simulink model "Mdl_Dim"  (R2024b)
settings: Solver=FixedStepDiscrete  StartTime=0.0  StopTime=10.0  FixedStep=0.1  RelTol=1e-3  EnableMultiTasking=on
values from neighbouring files (symbols this model uses):
  DEFAULT_MODE = mpt.Parameter    [Mdl_Dim_DD.m]
  DEFAULT_STEP = mpt.Parameter    [Mdl_Dim_DD.m]
  Mdl_Dim_cTaskPeriod = mpt.Parameter    [Mdl_Dim_rte_types.m]
  RTE_E_MAX_AGE_EXCEEDED = mpt.Parameter    [Mdl_Dim_rte_types.m]
  RTE_E_NEVER_RECEIVED = mpt.Parameter    [Mdl_Dim_rte_types.m]
  STATUS_OFF = mpt.Parameter    [Mdl_Dim_DD.m]
  STATUS_ON = mpt.Parameter    [Mdl_Dim_DD.m]
  SWITCHING_MECHANISM = mpt.Parameter    [Mdl_Dim_DD.m]
  ZERO_VAL = mpt.Parameter    [Mdl_Dim_DD.m]
undefined symbols (not defined in the file or in its folder): AppModule, CAN_COMUN_ACTIVE, CAN_COMUN_FAIL, CAN_VAL_OFF, CAN_VAL_ON, ChannelID, CLUSTER_ACTIVE, DAYNIGHT_STS_NOTRequire, DIAG_NCTRL, DIM_DAY_MODE, DIM_NIGHT_MODE, DOWN_THRESH_1SW, DrvRec_Rheo_down_Long_Press, DrvRec_Rheo_down_Short_Press, DrvRec_Rheo_up_Long_Press, DrvRec_Rheo_Up_Short_Press, DW_EVENT, DW_ON, eAppMdl_type_instance, eDayNightModeIn, eIllumination_levelIn, eSIGNAL_MISSING, eSIGNAL_NEVER_RECEIVED, eSleepSt_type_instance, FALSE, GetPwmDirect, GetPwmWithTime, GetPwmWithTimeExp, IgnOn, INDEX_MCUID0340, INDEX_MCUID0341, INDEX_MCUID0430, IoHwAb_PwmSignalIdType_type_instance, l_Wheel_Down_ParamArray, l_Wheel_Up_ParamArray, MAX_UINT16, MAXHOLD, MINHOLD, NETWORK_NORMAL, NETWORK_SLEEP, NETWORK_STANDALONE, NONE, NVM_Adapter_SetNVM_RheostatDayStep, NVM_Adapter_SetNVM_RheostatDayStepU1, NVM_Adapter_SetNVM_RheostatDayStepU2, NVM_Adapter_SetNVM_RheostatDayStepU3, NVM_Adapter_SetNVM_RheostatNightStep, NVM_Adapter_SetNVM_RheostatNightStepU1, NVM_Adapter_SetNVM_RheostatNightStepU2, NVM_Adapter_SetNVM_RheostatNightStepU3, OpeModeRheostatChange, pJustRcvdStatus, pNvmData, POS_MAX, POS_MIN, RHEO_1SW_TYPE, RHEO_2SW_TYPE, RHEO_SOFTSW_TYPE, RHEO_VALUE_FIVE_U16, RHEO_VALUE_ONE_BOOL ... (+48)
libraries: simulink x65
(part 3 of 4)

== system Mdl_Dim/Mdl_Dim_Task_sys/Subsystem/Input_Process/Switch Type//2 Switch Type//Soft Switch Type/RHEO_1SW_TYPE_AND_RHEO_2SW_TYPE/Subsystem2 ==
  ADC_RHDW_val : Inport
  AND : Logic  AllPortsSameDT=off  OutDataTypeStr=boolean
  Compare To Constant : simulink/Logic and Bit Operations/Compare To Constant  relop=~=  const=RHEO_VALUE_ZERO_BOOL  OutDataTypeStr=boolean
  Compare To Constant1 : simulink/Logic and Bit Operations/Compare To Constant  relop=~=  const=RHEO_VALUE_ONE_BOOL  OutDataTypeStr=boolean
  Compare To Constant5 : simulink/Logic and Bit Operations/Compare To Constant  relop===  const=RHEO_VALUE_ONE_BOOL  OutDataTypeStr=boolean
  Constant4 : Constant  Value=RHEO_VALUE_ONE_U16  OutDataTypeStr=Inherit: Inherit via back propagation
  Constant5 : Constant  Value=RHEO_VALUE_ZERO_U16  OutDataTypeStr=Inherit: Inherit via back propagation
  Constant6 : Constant  Value=RHEO_VALUE_ZERO_U16  OutDataTypeStr=uint16
  Constant7 : Constant  Value=RHEO_VALUE_FIVE_U16  OutDataTypeStr=Inherit: Inherit via back propagation
  Subtract1 : Sum  Inputs=+-
  Switch2 : Switch  Criteria=u2 ~= 0  OutDataTypeStr=uint16  SaturateOnIntegerOverflow=off  InputSameDT=off
  Switch3 : Switch  Criteria=u2 ~= 0  OutDataTypeStr=uint16  RndMeth=Simplest  SaturateOnIntegerOverflow=off  InputSameDT=off
  Unit Delay : UnitDelay  SampleTime=-1  StateName=Prev_RHDW_RawIn_Val  HasFrameUpgradeWarning=on
  Unit Delay2 : UnitDelay  InitialCondition=ZERO_DUTY  SampleTime=-1  StateName=Prev_SW1Rheostat_Dw_time_Step50ms  HasFrameUpgradeWarning=on
  check count2 : RelationalOperator  Operator=~=  OutDataTypeStr=boolean  InputSameDT=off
  RHDW_RawIn_Val_50ms : Outport  VectorParamsAs1DForOutWhenUnconnected=off
  wires:
  Unit Delay2/1 -> Switch2/3  "current_count_2"
  Switch2/1 -> Subtract1/1, check count2/1  "current_count_2"
  check count2/1 -> RHDW_RawIn_Val_50ms/1, Switch3/2  "fl_RHDW_RawIn_Val_50ms"
  Compare To Constant5/1 -> Switch2/2
  Constant4/1 -> Subtract1/2  "Decrement_Value_2"
  Constant7/1 -> Switch2/1  "Decrement_Value_DW"
  Switch3/1 -> Unit Delay2/1
  Constant5/1 -> check count2/2  "Max_step_Count2"
  ADC_RHDW_val/1 -> [RHDW_RawIn_Val], Unit Delay/1
  Unit Delay/1 -> [Prev_RHDW_RawIn_Val]
  [RHDW_RawIn_Val] -> Compare To Constant/1
  [Prev_RHDW_RawIn_Val] -> Compare To Constant1/1
  Constant6/1 -> Switch3/3
  Subtract1/1 -> Switch3/1  "current_count_2"
  Compare To Constant/1 -> AND/1
  Compare To Constant1/1 -> AND/2
  AND/1 -> Compare To Constant5/1

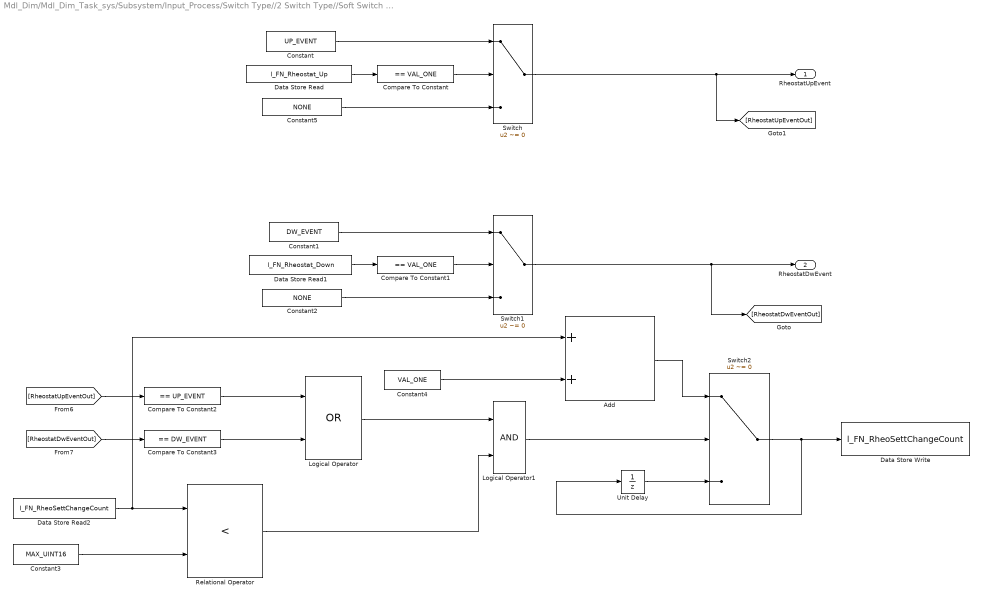
== system Mdl_Dim/Mdl_Dim_Task_sys/Subsystem/Input_Process/Switch Type//2 Switch Type//Soft Switch Type/Soft Switch Type/Event Check ==
  Add : Sum
  Compare To Constant : simulink/Logic and Bit Operations/Compare To Constant  relop===  const=VAL_ONE  OutDataTypeStr=boolean
  Compare To Constant1 : simulink/Logic and Bit Operations/Compare To Constant  relop===  const=VAL_ONE  OutDataTypeStr=boolean
  Compare To Constant2 : simulink/Logic and Bit Operations/Compare To Constant  relop===  const=UP_EVENT  OutDataTypeStr=boolean
  Compare To Constant3 : simulink/Logic and Bit Operations/Compare To Constant  relop===  const=DW_EVENT  OutDataTypeStr=boolean
  Constant : Constant  Value=UP_EVENT
  Constant1 : Constant  Value=DW_EVENT
  Constant2 : Constant  Value=NONE
  Constant3 : Constant  Value=MAX_UINT16  OutDataTypeStr=uint16
  Constant4 : Constant  Value=VAL_ONE  OutDataTypeStr=uint16
  Constant5 : Constant  Value=NONE
  Data Store Read : DataStoreRead  DataStoreName=l_FN_Rheostat_Up  IndexOptions=Index vector (dialog)  Indices=1  OutputSizes=1
  Data Store Read1 : DataStoreRead  DataStoreName=l_FN_Rheostat_Down  IndexOptions=Index vector (dialog)  Indices=1  OutputSizes=1
  Data Store Read2 : DataStoreRead  DataStoreName=l_FN_RheoSettChangeCount  IndexOptions=Index vector (dialog)  Indices=1  OutputSizes=1
  Data Store Write : DataStoreWrite  DataStoreName=l_FN_RheoSettChangeCount  IndexOptions=Index vector (dialog)  Indices=1  OutputSizes=1
  Logical Operator : Logic  Operator=OR  AllPortsSameDT=off  OutDataTypeStr=boolean
  Logical Operator1 : Logic  AllPortsSameDT=off  OutDataTypeStr=boolean
  Relational Operator : RelationalOperator  Operator=<  OutDataTypeStr=boolean  RndMeth=Simplest  InputSameDT=off
  Switch : Switch  Criteria=u2 ~= 0  SaturateOnIntegerOverflow=off  InputSameDT=off
  Switch1 : Switch  Criteria=u2 ~= 0  SaturateOnIntegerOverflow=off  InputSameDT=off
  Switch2 : Switch  Criteria=u2 ~= 0  SaturateOnIntegerOverflow=off  InputSameDT=off
  Unit Delay : UnitDelay  SampleTime=-1  HasFrameUpgradeWarning=on
  RheostatUpEvent : Outport  VectorParamsAs1DForOutWhenUnconnected=off
  RheostatDwEvent : Outport  Port=2  VectorParamsAs1DForOutWhenUnconnected=off
  wires:
  Compare To Constant1/1 -> Switch1/2
  Constant/1 -> Switch/1
  Data Store Read1/1 -> Compare To Constant1/1
  Data Store Read/1 -> Compare To Constant/1
  Constant1/1 -> Switch1/1
  Compare To Constant/1 -> Switch/2
  Constant2/1 -> Switch1/3
  Constant5/1 -> Switch/3
  Switch1/1 -> [RheostatDwEventOut], RheostatDwEvent/1
  Switch/1 -> [RheostatUpEventOut], RheostatUpEvent/1
  Switch2/1 -> Unit Delay/1, Data Store Write/1
  Data Store Read2/1 -> Add/1, Relational Operator/1
  [RheostatDwEventOut] -> Compare To Constant3/1
  Constant4/1 -> Add/2
  Relational Operator/1 -> Logical Operator1/2
  Unit Delay/1 -> Switch2/3
  Logical Operator/1 -> Logical Operator1/1
  Constant3/1 -> Relational Operator/2
  Add/1 -> Switch2/1
  [RheostatUpEventOut] -> Compare To Constant2/1
  Compare To Constant2/1 -> Logical Operator/1
  Compare To Constant3/1 -> Logical Operator/2
  Logical Operator1/1 -> Switch2/2

== system Mdl_Dim/Mdl_Dim_Task_sys/Subsystem/Input_Process/Switch Type//2 Switch Type//Soft Switch Type/Soft Switch Type/Event Clear ==
  Constant3 : Constant  Value=NONE
  Constant4 : Constant  Value=NONE
  Data Store Write : DataStoreWrite  DataStoreName=l_FN_Rheostat_Up  IndexOptions=Index vector (dialog)  Indices=1  OutputSizes=1
  Data Store Write1 : DataStoreWrite  DataStoreName=l_FN_Rheostat_Down  IndexOptions=Index vector (dialog)  Indices=1  OutputSizes=1
  wires:
  Constant3/1 -> Data Store Write/1
  Constant4/1 -> Data Store Write1/1

== system Mdl_Dim/Mdl_Dim_Task_sys/Subsystem/Input_Process/Switch Type//2 Switch Type//Soft Switch Type/Subsystem1/If Action Subsystem ==
  Action Port : ActionPort
  Constant : Constant  Value=VAL_ON
  Data Store Read1 : DataStoreRead  DataStoreName=l_Prev_NVM_RheostatNightStep  IndexOptions=Index vector (dialog)  Indices=1  OutputSizes=1
  Data Store Read2 : DataStoreRead  DataStoreName=l_Prev_NVM_RheostatDayStep  IndexOptions=Index vector (dialog)  Indices=1  OutputSizes=1
  NVM_Adapter_SetNVM_RheostatDayStep : FunctionCaller  FunctionPrototype=NVM_Adapter_SetNVM_RheostatDayStep(pNvmData)  InputArgumentSpecifications=uint8(1)  OutputArgumentSpecifications=<Enter example>
  NVM_Adapter_SetNVM_RheostatNightStep : FunctionCaller  FunctionPrototype=NVM_Adapter_SetNVM_RheostatNightStep(pNvmData)  InputArgumentSpecifications=uint8(1)  OutputArgumentSpecifications=<Enter example>
  OpeModeRheostatChange : FunctionCaller  FunctionPrototype=OpeModeRheostatChange()  InputArgumentSpecifications=<Enter example>  OutputArgumentSpecifications=<Enter example>
  RheostatChange : Outport  VectorParamsAs1DForOutWhenUnconnected=off
  wires:
  Constant/1 -> RheostatChange/1
  Data Store Read1/1 -> NVM_Adapter_SetNVM_RheostatNightStep/1
  Data Store Read2/1 -> NVM_Adapter_SetNVM_RheostatDayStep/1

== system Mdl_Dim/Mdl_Dim_Task_sys/Subsystem/Input_Process/Switch Type//2 Switch Type//Soft Switch Type/Subsystem1/If Action Subsystem1 ==
  Action Port : ActionPort
  Constant : Constant  Value=VAL_OFF
  RheostatChange : Outport  VectorParamsAs1DForOutWhenUnconnected=off
  wires:
  Constant/1 -> RheostatChange/1

== system Mdl_Dim/Mdl_Dim_Task_sys/Subsystem/Input_Process/Thumb Wheel Type/Rheostat_ONS_Status_Output /Debounce_timer_Subsystem2 ==
  Debounce_Count : Inport
  "ResetTimerStatus " : Inport  Port=2
  Compare To Zero : simulink/Logic and Bit Operations/Compare To Zero  relop=~=  OutDataTypeStr=boolean
  Compare To Zero1 : simulink/Logic and Bit Operations/Compare To Zero  relop=~=  OutDataTypeStr=boolean
  Constant1 : Constant  Value=VAL_ONE  OutDataTypeStr=uint8
  Constant2 : Constant  Value=VAL_ONE  OutDataTypeStr=uint8
  Constant3 : Constant  Value=VAL_ZERO  OutDataTypeStr=uint8
  Constant4 : Constant  Value=VAL_ZERO  OutDataTypeStr=uint8
  Data Store Read : DataStoreRead  DataStoreName=l_Prev_Rheo3secCount  IndexOptions=Index vector (dialog)  Indices=1  OutputSizes=1
  Data Store Read1 : DataStoreRead  DataStoreName=l_Prev_Rheo3secCount  IndexOptions=Index vector (dialog)  Indices=1  OutputSizes=1
  Data Store Write : DataStoreWrite  DataStoreName=l_Prev_Rheo3secCount  IndexOptions=Index vector (dialog)  Indices=1  OutputSizes=1
  Sum : Sum
  Switch1 : Switch  Criteria=u2 ~= 0  OutDataTypeStr=uint32  SaturateOnIntegerOverflow=off  InputSameDT=off
  Switch2 : Switch  Criteria=u2 ~= 0  OutDataTypeStr=uint32  SaturateOnIntegerOverflow=off  InputSameDT=off
  Switch3 : Switch  Criteria=u2 ~= 0  OutDataTypeStr=uint32  SaturateOnIntegerOverflow=off  InputSameDT=off
  check count1 : RelationalOperator  Operator=<=  OutDataTypeStr=boolean  InputSameDT=off
  wires:
  "ResetTimerStatus "/1 -> Compare To Zero/1
  Switch2/1 -> Switch3/3, check count1/2  "current_count"
  Debounce_Count/1 -> check count1/1  "debounce_count"
  check count1/1 -> Switch3/2  "debounce_status"
  Constant2/1 -> Switch2/1
  Compare To Zero/1 -> Switch2/2
  Constant1/1 -> Sum/1
  Data Store Read/1 -> Sum/2
  Data Store Read1/1 -> Compare To Zero1/1
  Compare To Zero1/1 -> Switch1/2
  Switch1/1 -> Switch2/3
  Sum/1 -> Switch1/1
  Constant3/1 -> Switch1/3
  Switch3/1 -> Data Store Write/1
  Constant4/1 -> Switch3/1

== system Mdl_Dim/Mdl_Dim_Task_sys/Subsystem/Input_Process/Thumb Wheel Type/Rheostat_ONS_Status_Output /Subsystem3 ==
  Action Port : ActionPort
  Constant : Constant  Value=VAL_ONE
  Data Store Write : DataStoreWrite  DataStoreName=RheostatONSStatus  IndexOptions=Index vector (dialog)  Indices=1  OutputSizes=1
  wires:
  Constant/1 -> Data Store Write/1

== system Mdl_Dim/Mdl_Dim_Task_sys/Subsystem/Input_Process/Thumb Wheel Type/Rheostat_ONS_Status_Output /Subsystem4 ==
  Action Port : ActionPort
  Constant1 : Constant  Value=VAL_TWO
  Data Store Write : DataStoreWrite  DataStoreName=RheostatONSStatus  IndexOptions=Index vector (dialog)  Indices=1  OutputSizes=1
  wires:
  Constant1/1 -> Data Store Write/1

== system Mdl_Dim/Mdl_Dim_Task_sys/Subsystem/Input_Process/Thumb Wheel Type/Rheostat_ONS_Status_Output /Subsystem5 ==
  Action Port : ActionPort
  Constant1 : Constant  Value=VAL_ZERO
  Data Store Read : DataStoreRead  DataStoreName=RheostatONSStatus  IndexOptions=Index vector (dialog)  Indices=1  OutputSizes=1
  Data Store Read1 : DataStoreRead  DataStoreName=l_Prev_Rheo3secCount  IndexOptions=Index vector (dialog)  Indices=1  OutputSizes=1
  Data Store Write : DataStoreWrite  DataStoreName=RheostatONSStatus  IndexOptions=Index vector (dialog)  Indices=1  OutputSizes=1
  Switch : Switch  Criteria=u2 ~= 0  SaturateOnIntegerOverflow=off  InputSameDT=off
  wires:
  Data Store Read1/1 -> Switch/2
  Constant1/1 -> Switch/3
  Switch/1 -> Data Store Write/1
  Data Store Read/1 -> Switch/1

== system Mdl_Dim/Mdl_Dim_Task_sys/Subsystem/Input_Process/Thumb Wheel Type/Subsystem/Subsystem1 ==
  RHEO_SW_WHEEL : Inport
  ADC_RHEO_5V_MON_ADI : Inport  Port=2
  Compare To Constant : simulink/Logic and Bit Operations/Compare To Constant  relop=>=  const=WHEELVOLRATIO_SAMPLE_COUNT  OutDataTypeStr=boolean
  Data Store Read1 : DataStoreRead  DataStoreName=l_Wheel_Vol_Counter_u8  IndexOptions=Index vector (dialog)  Indices=1  OutputSizes=1
  Enabled Subsystem : Subsystem  TreatAsAtomicUnit=on
  Subsystem : Subsystem
  wires:
  Data Store Read1/1 -> Compare To Constant/1
  Compare To Constant/1 -> Enabled Subsystem/Enable
  ADC_RHEO_5V_MON_ADI/1 -> Subsystem/2(ADC_RHEO_5V_MON_ADI)
  RHEO_SW_WHEEL/1 -> Subsystem/1(RHEO_SW_WHEEL)

== system Mdl_Dim/Mdl_Dim_Task_sys/Subsystem/Input_Process/Switch Type//2 Switch Type//Soft Switch Type/RHEO_1SW_TYPE_AND_RHEO_2SW_TYPE/ Rheostat Dw  Event Determination/Enabled Subsystem ==
  Enable : EnablePort
  Constant : Constant  OutDataTypeStr=boolean
  DrvRec_Rheo_down_Long_Press : FunctionCaller  FunctionPrototype=DrvRec_Rheo_down_Long_Press(SWGrp4LongPress_Status)  InputArgumentSpecifications=boolean(1)  OutputArgumentSpecifications=<Enter example>
  wires:
  Constant/1 -> DrvRec_Rheo_down_Long_Press/1

== system Mdl_Dim/Mdl_Dim_Task_sys/Subsystem/Input_Process/Switch Type//2 Switch Type//Soft Switch Type/RHEO_1SW_TYPE_AND_RHEO_2SW_TYPE/ Rheostat Dw  Event Determination/Enabled Subsystem1 ==
  Enable : EnablePort
  Constant : Constant  OutDataTypeStr=boolean
  DrvRec_Rheo_down_Short_Press : FunctionCaller  FunctionPrototype=DrvRec_Rheo_down_Short_Press(SWGrp4ShortPress_Status)  InputArgumentSpecifications=boolean(1)  OutputArgumentSpecifications=<Enter example>
  wires:
  Constant/1 -> DrvRec_Rheo_down_Short_Press/1

== system Mdl_Dim/Mdl_Dim_Task_sys/Subsystem/Input_Process/Switch Type//2 Switch Type//Soft Switch Type/RHEO_1SW_TYPE_AND_RHEO_2SW_TYPE/ Rheostat Dw  Event Determination/Timer_100ms ==
  Debounce_Count : Inport
  "ResetTimerStatus " : Inport  Port=2
  Timer_In : Inport  Port=3
  Compare To Zero : simulink/Logic and Bit Operations/Compare To Zero  relop===  OutDataTypeStr=boolean
  Constant1 : Constant  Value=VAL_ONE  OutDataTypeStr=uint8
  Constant2 : Constant  Value=VAL_ZERO  OutDataTypeStr=uint8
  OR : Logic  Operator=OR  AllPortsSameDT=off  OutDataTypeStr=boolean
  Sum : Sum
  Switch2 : Switch  Criteria=u2 ~= 0  OutDataTypeStr=uint16  SaturateOnIntegerOverflow=off  InputSameDT=off
  check count1 : RelationalOperator  Operator=<=  OutDataTypeStr=boolean  InputSameDT=off
  TimerDebouncestatus : Outport  VectorParamsAs1DForOutWhenUnconnected=off
  Timer_out : Outport  Port=2  VectorParamsAs1DForOutWhenUnconnected=off
  wires:
  "ResetTimerStatus "/1 -> Compare To Zero/1
  Constant2/1 -> Switch2/1
  Sum/1 -> Switch2/3, check count1/2
  Constant1/1 -> Sum/1
  check count1/1 -> OR/2, TimerDebouncestatus/1  "debounce_status"
  Debounce_Count/1 -> [Debounce_Count]  "debounce_count"
  [Debounce_Count] -> check count1/1
  Compare To Zero/1 -> OR/1
  OR/1 -> Switch2/2
  Switch2/1 -> Timer_out/1  "current_count"
  Timer_In/1 -> Sum/2

== system Mdl_Dim/Mdl_Dim_Task_sys/Subsystem/Input_Process/Switch Type//2 Switch Type//Soft Switch Type/RHEO_1SW_TYPE_AND_RHEO_2SW_TYPE/ Rheostat Dw  Event Determination/Timer_800ms ==
  Debounce_Count : Inport
  "ResetTimerStatus " : Inport  Port=2
  l_PrevTimerSt_In : Inport  Port=3
  AND : Logic  AllPortsSameDT=off  OutDataTypeStr=boolean
  Constant1 : Constant  Value=VAL_ONE  OutDataTypeStr=uint8
  Constant2 : Constant  Value=VAL_ZERO  OutDataTypeStr=uint8
  Constant3 : Constant  Value=VAL_ZERO  OutDataTypeStr=uint8
  Sum : Sum
  Switch2 : Switch  Criteria=u2 ~= 0  OutDataTypeStr=uint32  SaturateOnIntegerOverflow=off  InputSameDT=off
  Switch3 : Switch  Criteria=u2 ~= 0  OutDataTypeStr=uint16  SaturateOnIntegerOverflow=off  InputSameDT=off
  check count : RelationalOperator  OutDataTypeStr=boolean  InputSameDT=off
  check count1 : RelationalOperator  Operator=~=  OutDataTypeStr=boolean  InputSameDT=off
  check count2 : RelationalOperator  Operator=>  OutDataTypeStr=boolean  InputSameDT=off
  Timer_800ms_elapsed_status : Outport  VectorParamsAs1DForOutWhenUnconnected=off
  Timer_Running_Status : Outport  Port=2  VectorParamsAs1DForOutWhenUnconnected=off
  l_PrevTimerSt_Out : Outport  Port=3  VectorParamsAs1DForOutWhenUnconnected=off
  wires:
  "ResetTimerStatus "/1 -> Switch2/2
  Switch2/1 -> Switch3/3, check count/1  "current_count"
  Debounce_Count/1 -> check count/2, check count2/1, Switch3/1  "debounce_count"
  check count/1 -> Timer_800ms_elapsed_status/1, Switch3/2  "debounce_status"
  Switch3/1 -> l_PrevTimerSt_Out/1
  Constant2/1 -> Switch2/1
  Sum/1 -> Switch2/3
  l_PrevTimerSt_In/1 -> check count1/2, check count2/2, Sum/2
  Constant1/1 -> Sum/1
  Constant3/1 -> check count1/1
  check count2/1 -> AND/1  "debounce_status"
  check count1/1 -> AND/2  "debounce_status"
  AND/1 -> Timer_Running_Status/1

== system Mdl_Dim/Mdl_Dim_Task_sys/Subsystem/Input_Process/Switch Type//2 Switch Type//Soft Switch Type/RHEO_1SW_TYPE_AND_RHEO_2SW_TYPE/ Rheostat Up Event Determination/Enabled Subsystem ==
  Enable : EnablePort
  Constant : Constant  OutDataTypeStr=boolean
  DrvRec_Rheo_up_Long_Press : FunctionCaller  FunctionPrototype=DrvRec_Rheo_up_Long_Press(SWGrp4LongPress_Status)  InputArgumentSpecifications=boolean(1)  OutputArgumentSpecifications=<Enter example>
  wires:
  Constant/1 -> DrvRec_Rheo_up_Long_Press/1

== system Mdl_Dim/Mdl_Dim_Task_sys/Subsystem/Input_Process/Switch Type//2 Switch Type//Soft Switch Type/RHEO_1SW_TYPE_AND_RHEO_2SW_TYPE/ Rheostat Up Event Determination/Enabled Subsystem1 ==
  Enable : EnablePort
  Constant : Constant  OutDataTypeStr=boolean
  DrvRec_Rheo_Up_Short_Press : FunctionCaller  FunctionPrototype=DrvRec_Rheo_Up_Short_Press(SWGrp4ShortPress_Status)  InputArgumentSpecifications=boolean(1)  OutputArgumentSpecifications=<Enter example>
  wires:
  Constant/1 -> DrvRec_Rheo_Up_Short_Press/1

== system Mdl_Dim/Mdl_Dim_Task_sys/Subsystem/Input_Process/Switch Type//2 Switch Type//Soft Switch Type/RHEO_1SW_TYPE_AND_RHEO_2SW_TYPE/ Rheostat Up Event Determination/Timer_100ms ==
  Debounce_Count : Inport
  "ResetTimerStatus " : Inport  Port=2
  Timer_In : Inport  Port=3
  Compare To Zero : simulink/Logic and Bit Operations/Compare To Zero  relop===  OutDataTypeStr=boolean
  Constant1 : Constant  Value=VAL_ONE  OutDataTypeStr=uint8
  Constant2 : Constant  Value=VAL_ZERO  OutDataTypeStr=uint8
  OR : Logic  Operator=OR  AllPortsSameDT=off  OutDataTypeStr=boolean
  Sum : Sum
  Switch2 : Switch  Criteria=u2 ~= 0  OutDataTypeStr=uint16  SaturateOnIntegerOverflow=off  InputSameDT=off
  check count1 : RelationalOperator  Operator=<=  OutDataTypeStr=boolean  InputSameDT=off
  TimerDebouncestatus : Outport  VectorParamsAs1DForOutWhenUnconnected=off
  Timer_out : Outport  Port=2  VectorParamsAs1DForOutWhenUnconnected=off
  wires:
  "ResetTimerStatus "/1 -> Compare To Zero/1
  Constant2/1 -> Switch2/1
  Sum/1 -> Switch2/3, check count1/2
  Constant1/1 -> Sum/1
  check count1/1 -> OR/2, TimerDebouncestatus/1  "debounce_status"
  Debounce_Count/1 -> [Debounce_Count]  "debounce_count"
  [Debounce_Count] -> check count1/1
  Compare To Zero/1 -> OR/1
  OR/1 -> Switch2/2
  Switch2/1 -> Timer_out/1  "current_count"
  Timer_In/1 -> Sum/2

== system Mdl_Dim/Mdl_Dim_Task_sys/Subsystem/Input_Process/Switch Type//2 Switch Type//Soft Switch Type/RHEO_1SW_TYPE_AND_RHEO_2SW_TYPE/ Rheostat Up Event Determination/Timer_800ms ==
  Debounce_Count : Inport
  "ResetTimerStatus " : Inport  Port=2
  l_PrevTimerSt_In : Inport  Port=3
  AND : Logic  AllPortsSameDT=off  OutDataTypeStr=boolean
  Constant1 : Constant  Value=VAL_ONE  OutDataTypeStr=uint8
  Constant2 : Constant  Value=VAL_ZERO  OutDataTypeStr=uint8
  Constant3 : Constant  Value=VAL_ZERO  OutDataTypeStr=uint8
  Sum : Sum
  Switch2 : Switch  Criteria=u2 ~= 0  OutDataTypeStr=uint32  SaturateOnIntegerOverflow=off  InputSameDT=off
  Switch3 : Switch  Criteria=u2 ~= 0  OutDataTypeStr=uint16  SaturateOnIntegerOverflow=off  InputSameDT=off
  check count : RelationalOperator  OutDataTypeStr=boolean  InputSameDT=off
  check count1 : RelationalOperator  Operator=~=  OutDataTypeStr=boolean  InputSameDT=off
  check count2 : RelationalOperator  Operator=>  OutDataTypeStr=boolean  InputSameDT=off
  Timer_800ms_elapsed_status : Outport  VectorParamsAs1DForOutWhenUnconnected=off
  Timer_Running_Status : Outport  Port=2  VectorParamsAs1DForOutWhenUnconnected=off
  l_PrevTimerSt_Out : Outport  Port=3  VectorParamsAs1DForOutWhenUnconnected=off
  wires:
  "ResetTimerStatus "/1 -> Switch2/2
  Switch2/1 -> Switch3/3, check count/1  "current_count"
  Debounce_Count/1 -> check count/2, check count2/1, Switch3/1  "debounce_count"
  check count/1 -> Timer_800ms_elapsed_status/1, Switch3/2  "debounce_status"
  Switch3/1 -> l_PrevTimerSt_Out/1
  Constant2/1 -> Switch2/1
  Sum/1 -> Switch2/3
  l_PrevTimerSt_In/1 -> check count1/2, check count2/2, Sum/2
  Constant1/1 -> Sum/1
  Constant3/1 -> check count1/1
  check count2/1 -> AND/1  "debounce_status"
  check count1/1 -> AND/2  "debounce_status"
  AND/1 -> Timer_Running_Status/1

== system Mdl_Dim/Mdl_Dim_Task_sys/Subsystem/Input_Process/Switch Type//2 Switch Type//Soft Switch Type/RHEO_1SW_TYPE_AND_RHEO_2SW_TYPE/Rheostat_ONS_Status_Output /Debounce_timer_Subsystem2 ==
  Debounce_Count : Inport
  "ResetTimerStatus " : Inport  Port=2
  Compare To Zero : simulink/Logic and Bit Operations/Compare To Zero  relop=~=  OutDataTypeStr=boolean
  Compare To Zero1 : simulink/Logic and Bit Operations/Compare To Zero  relop=~=  OutDataTypeStr=boolean
  Constant1 : Constant  Value=VAL_ONE  OutDataTypeStr=uint8
  Constant2 : Constant  Value=VAL_ONE  OutDataTypeStr=uint8
  Constant3 : Constant  Value=VAL_ZERO  OutDataTypeStr=uint8
  Constant4 : Constant  Value=VAL_ZERO  OutDataTypeStr=uint8
  Data Store Read : DataStoreRead  DataStoreName=l_Prev_Rheo3secCount  IndexOptions=Index vector (dialog)  Indices=1  OutputSizes=1
  Data Store Read1 : DataStoreRead  DataStoreName=l_Prev_Rheo3secCount  IndexOptions=Index vector (dialog)  Indices=1  OutputSizes=1
  Data Store Write : DataStoreWrite  DataStoreName=l_Prev_Rheo3secCount  IndexOptions=Index vector (dialog)  Indices=1  OutputSizes=1
  Sum : Sum
  Switch1 : Switch  Criteria=u2 ~= 0  OutDataTypeStr=uint32  SaturateOnIntegerOverflow=off  InputSameDT=off
  Switch2 : Switch  Criteria=u2 ~= 0  OutDataTypeStr=uint32  SaturateOnIntegerOverflow=off  InputSameDT=off
  Switch3 : Switch  Criteria=u2 ~= 0  OutDataTypeStr=uint32  SaturateOnIntegerOverflow=off  InputSameDT=off
  check count1 : RelationalOperator  Operator=<=  OutDataTypeStr=boolean  InputSameDT=off
  wires:
  "ResetTimerStatus "/1 -> Compare To Zero/1
  Switch2/1 -> Switch3/3, check count1/2  "current_count"
  Debounce_Count/1 -> check count1/1  "debounce_count"
  check count1/1 -> Switch3/2  "debounce_status"
  Constant2/1 -> Switch2/1
  Compare To Zero/1 -> Switch2/2
  Constant1/1 -> Sum/1
  Data Store Read/1 -> Sum/2
  Data Store Read1/1 -> Compare To Zero1/1
  Compare To Zero1/1 -> Switch1/2
  Switch1/1 -> Switch2/3
  Sum/1 -> Switch1/1
  Constant3/1 -> Switch1/3
  Switch3/1 -> Data Store Write/1
  Constant4/1 -> Switch3/1

== system Mdl_Dim/Mdl_Dim_Task_sys/Subsystem/Input_Process/Switch Type//2 Switch Type//Soft Switch Type/RHEO_1SW_TYPE_AND_RHEO_2SW_TYPE/Rheostat_ONS_Status_Output /Subsystem3 ==
  Action Port : ActionPort
  Constant : Constant  Value=VAL_ONE
  Data Store Write : DataStoreWrite  DataStoreName=RheostatONSStatus  IndexOptions=Index vector (dialog)  Indices=1  OutputSizes=1
  wires:
  Constant/1 -> Data Store Write/1

== system Mdl_Dim/Mdl_Dim_Task_sys/Subsystem/Input_Process/Switch Type//2 Switch Type//Soft Switch Type/RHEO_1SW_TYPE_AND_RHEO_2SW_TYPE/Rheostat_ONS_Status_Output /Subsystem4 ==
  Action Port : ActionPort
  Constant1 : Constant  Value=VAL_TWO
  Data Store Write : DataStoreWrite  DataStoreName=RheostatONSStatus  IndexOptions=Index vector (dialog)  Indices=1  OutputSizes=1
  wires:
  Constant1/1 -> Data Store Write/1

== system Mdl_Dim/Mdl_Dim_Task_sys/Subsystem/Input_Process/Switch Type//2 Switch Type//Soft Switch Type/RHEO_1SW_TYPE_AND_RHEO_2SW_TYPE/Rheostat_ONS_Status_Output /Subsystem5 ==
  Action Port : ActionPort
  Constant1 : Constant  Value=VAL_ZERO
  Data Store Read : DataStoreRead  DataStoreName=RheostatONSStatus  IndexOptions=Index vector (dialog)  Indices=1  OutputSizes=1
  Data Store Read1 : DataStoreRead  DataStoreName=l_Prev_Rheo3secCount  IndexOptions=Index vector (dialog)  Indices=1  OutputSizes=1
  Data Store Write : DataStoreWrite  DataStoreName=RheostatONSStatus  IndexOptions=Index vector (dialog)  Indices=1  OutputSizes=1
  Switch : Switch  Criteria=u2 ~= 0  SaturateOnIntegerOverflow=off  InputSameDT=off
  wires:
  Data Store Read1/1 -> Switch/2
  Constant1/1 -> Switch/3
  Switch/1 -> Data Store Write/1
  Data Store Read/1 -> Switch/1

== system Mdl_Dim/Mdl_Dim_Task_sys/Subsystem/Input_Process/Thumb Wheel Type/Subsystem/Subsystem1/Enabled Subsystem ==
  Enable : EnablePort
  Average : Subsystem  Priority=1
      settings: AttributesFormatString=Priority = %<Priority>
  Reinit : Subsystem  Priority=2
      settings: AttributesFormatString=Priority = %<Priority>

== system Mdl_Dim/Mdl_Dim_Task_sys/Subsystem/Input_Process/Thumb Wheel Type/Subsystem/Subsystem1/Subsystem ==
  RHEO_SW_WHEEL : Inport  OutDataTypeStr=uint16
  ADC_RHEO_5V_MON_ADI : Inport  Port=2  OutDataTypeStr=uint16
  Add : Sum
  Add1 : Sum
  Constant : Constant  Value=WHEELVOLRATIO_100PER
  Constant1 : Constant  Value=WHEELVOLRATIO_100PER
  Constant2 : Constant  Value=VAL_ONE
  Data Store Read : DataStoreRead  DataStoreName=l_Wheel_Vol_Counter_u8  IndexOptions=Index vector (dialog)  Indices=1  OutputSizes=1
  Data Store Read2 : DataStoreRead  DataStoreName=l_Wheel_BuffVol_u32  IndexOptions=Index vector (dialog)  Indices=1  OutputSizes=1
  Data Store Write : DataStoreWrite  DataStoreName=l_Wheel_Vol_Counter_u8  IndexOptions=Index vector (dialog)  Indices=1  OutputSizes=1
  Data Store Write1 : DataStoreWrite  DataStoreName=l_Wheel_BuffVol_u32  IndexOptions=Index vector (dialog)  Indices=1  OutputSizes=1
  Divide : Product  Inputs=*/  OutDataTypeStr=uint16
  GreaterThan : RelationalOperator  OutDataTypeStr=boolean  RndMeth=Simplest  InputSameDT=off
  Multiply : Product  OutDataTypeStr=uint32
  Switch : Switch  Criteria=u2 ~= 0  SaturateOnIntegerOverflow=off  InputSameDT=off
  wires:
  Divide/1 -> Switch/3
  Data Store Read2/1 -> Add1/2
  Multiply/1 -> Divide/1
  GreaterThan/1 -> Switch/2
  Constant/1 -> Switch/1
  [ADC_RHEO_5V_MON_ADI] -> Divide/2
  Add1/1 -> Data Store Write1/1
  [RHEO_SW_WHEEL] -> Multiply/1
  Switch/1 -> Add1/1
  Constant1/1 -> Multiply/2
  ADC_RHEO_5V_MON_ADI/1 -> [ADC_RHEO_5V_MON_ADI]
  RHEO_SW_WHEEL/1 -> [RHEO_SW_WHEEL]
  Data Store Read/1 -> Add/1
  Add/1 -> Data Store Write/1
  Constant2/1 -> Add/2
  [RHEO_SW_WHEEL] -> GreaterThan/1
  [ADC_RHEO_5V_MON_ADI] -> GreaterThan/2

== system Mdl_Dim/Mdl_Dim_Task_sys/Subsystem/Input_Process/Thumb Wheel Type/Subsystem/Subsystem1/Enabled Subsystem/Average ==
  Compare To Constant1 : simulink/Logic and Bit Operations/Compare To Constant  relop===  const=WHEELVOLRATIO_100PER  OutDataTypeStr=boolean
  Data Store Read1 : DataStoreRead  DataStoreName=l_Wheel_BuffVol_u32  IndexOptions=Index vector (dialog)  Indices=1  OutputSizes=1
  Data Store Read2 : DataStoreRead  DataStoreName=l_Wheel_Vol_Counter_u8  IndexOptions=Index vector (dialog)  Indices=1  OutputSizes=1
  Data Store Read6 : DataStoreRead  DataStoreName=l_Wheel_AveVol_u32  IndexOptions=Index vector (dialog)  Indices=1  OutputSizes=1
  Data Store Write : DataStoreWrite  DataStoreName=l_Wheel_AveVol_u32  IndexOptions=Index vector (dialog)  Indices=1  OutputSizes=1
  Divide : Product  Inputs=*/  OutDataTypeStr=uint32
  If : If  IfExpression=u1 ~= 0
  If Action Subsystem : Subsystem  TreatAsAtomicUnit=on
  Subsystem : Subsystem
  wires:
  Divide/1 -> Data Store Write/1
  Data Store Read2/1 -> Divide/2
  Data Store Read1/1 -> Divide/1
  Data Store Read6/1 -> Compare To Constant1/1
  Compare To Constant1/1 -> If/1
  If/1 -> If Action Subsystem/Action
  If/2 -> Subsystem/Action

== system Mdl_Dim/Mdl_Dim_Task_sys/Subsystem/Input_Process/Thumb Wheel Type/Subsystem/Subsystem1/Enabled Subsystem/Reinit ==
  Constant : Constant  Value=VAL_OFF
  Constant1 : Constant  Value=RHEO_VALUE_ZERO_U32
  Data Store Write1 : DataStoreWrite  DataStoreName=l_Wheel_Vol_Counter_u8  IndexOptions=Index vector (dialog)  Indices=1  OutputSizes=1
  Data Store Write2 : DataStoreWrite  DataStoreName=l_Wheel_BuffVol_u32  IndexOptions=Index vector (dialog)  Indices=1  OutputSizes=1
  wires:
  Constant/1 -> Data Store Write1/1
  Constant1/1 -> Data Store Write2/1

== system Mdl_Dim/Mdl_Dim_Task_sys/Subsystem/Input_Process/Thumb Wheel Type/Subsystem/Subsystem1/Enabled Subsystem/Average/If Action Subsystem ==
  Action Port : ActionPort
  Constant : Constant  Value=POS_MAX
  Data Store Write1 : DataStoreWrite  DataStoreName=l_Wheel_Position_Temp_u8  IndexOptions=Index vector (dialog)  Indices=1  OutputSizes=1
  wires:
  Constant/1 -> Data Store Write1/1

== system Mdl_Dim/Mdl_Dim_Task_sys/Subsystem/Input_Process/Thumb Wheel Type/Subsystem/Subsystem1/Enabled Subsystem/Average/Subsystem ==
  Action Port : ActionPort
  Data Store Read : DataStoreRead  DataStoreName=l_Wheel_AveVol_u32  IndexOptions=Index vector (dialog)  Indices=1  OutputSizes=1
  Data Store Read3 : DataStoreRead  DataStoreName=l_Positionthreshhold_Down  IndexOptions=Index vector (dialog)  Indices=1  OutputSizes=1
  Data Store Read4 : DataStoreRead  DataStoreName=l_Positionthreshhold_Up  IndexOptions=Index vector (dialog)  Indices=1  OutputSizes=1
  Data Store Read5 : DataStoreRead  DataStoreName=l_Wheel_AveVol_u32  IndexOptions=Index vector (dialog)  Indices=1  OutputSizes=1
  Enabled Subsystem : Subsystem  TreatAsAtomicUnit=on
  GreaterThan : RelationalOperator  OutDataTypeStr=boolean  RndMeth=Simplest  InputSameDT=off
  GreaterThan1 : RelationalOperator  Operator=<=  OutDataTypeStr=boolean  RndMeth=Simplest  InputSameDT=off
  OR : Logic  Operator=OR  AllPortsSameDT=off  OutDataTypeStr=boolean
  wires:
  Data Store Read4/1 -> GreaterThan/2
  Data Store Read5/1 -> GreaterThan1/1
  Data Store Read/1 -> GreaterThan/1
  GreaterThan1/1 -> OR/2
  Data Store Read3/1 -> GreaterThan1/2
  OR/1 -> Enabled Subsystem/Enable
  GreaterThan/1 -> OR/1

== system Mdl_Dim/Mdl_Dim_Task_sys/Subsystem/Input_Process/Thumb Wheel Type/Subsystem/Subsystem1/Enabled Subsystem/Average/Subsystem/Enabled Subsystem ==
  Enable : EnablePort
  Data Store Read : DataStoreRead  DataStoreName=l_Wheel_AveVol_u32  IndexOptions=Index vector (dialog)  Indices=1  OutputSizes=1
  Data Store Read4 : DataStoreRead  DataStoreName=l_Positionthreshhold_Up  IndexOptions=Index vector (dialog)  Indices=1  OutputSizes=1
  GreaterThan : RelationalOperator  OutDataTypeStr=boolean  RndMeth=Simplest  InputSameDT=off
  If : If  IfExpression=u1 ~= 0
  If Action Subsystem : Subsystem  TreatAsAtomicUnit=on
  If Action Subsystem1 : Subsystem  TreatAsAtomicUnit=on
  wires:
  Data Store Read4/1 -> GreaterThan/2
  Data Store Read/1 -> GreaterThan/1
  GreaterThan/1 -> If/1
  If/1 -> If Action Subsystem/Action
  If/2 -> If Action Subsystem1/Action

== system Mdl_Dim/Mdl_Dim_Task_sys/Subsystem/Input_Process/Thumb Wheel Type/Subsystem/Subsystem1/Enabled Subsystem/Average/Subsystem/Enabled Subsystem/If Action Subsystem ==
  Action Port : ActionPort
  Compare To Constant : simulink/Logic and Bit Operations/Compare To Constant  relop=<  const=POS_MAX  OutDataTypeStr=boolean
  Data Store Read2 : DataStoreRead  DataStoreName=l_Wheel_Position_u8  IndexOptions=Index vector (dialog)  Indices=1  OutputSizes=1
  If : If  IfExpression=u1~=0  ShowElse=off
  If Action Subsystem1 : Subsystem  TreatAsAtomicUnit=on
  wires:
  If/1 -> If Action Subsystem1/Action
  Data Store Read2/1 -> Compare To Constant/1
  Compare To Constant/1 -> If/1

== system Mdl_Dim/Mdl_Dim_Task_sys/Subsystem/Input_Process/Thumb Wheel Type/Subsystem/Subsystem1/Enabled Subsystem/Average/Subsystem/Enabled Subsystem/If Action Subsystem1 ==
  Action Port : ActionPort
  Compare To Constant1 : simulink/Logic and Bit Operations/Compare To Constant  relop=>  const=POS_MIN  OutDataTypeStr=boolean
  Data Store Read2 : DataStoreRead  DataStoreName=l_Wheel_Position_u8  IndexOptions=Index vector (dialog)  Indices=1  OutputSizes=1
  If : If  IfExpression=u1~=0  ShowElse=off
  Subsystem : Subsystem
  wires:
  Data Store Read2/1 -> Compare To Constant1/1
  Compare To Constant1/1 -> If/1
  If/1 -> Subsystem/Action

== system Mdl_Dim/Mdl_Dim_Task_sys/Subsystem/Input_Process/Thumb Wheel Type/Subsystem/Subsystem1/Enabled Subsystem/Average/Subsystem/Enabled Subsystem/If Action Subsystem/If Action Subsystem1 ==
  Action Port : ActionPort
  Increament_Wheel : Subsystem  Priority=1
      settings: AttributesFormatString=Priority = %<Priority>
  Selecting_threshold : Subsystem  Priority=2
      settings: AttributesFormatString=Priority = %<Priority>  RTWFcnNameOpts=Use subsystem name

== system Mdl_Dim/Mdl_Dim_Task_sys/Subsystem/Input_Process/Thumb Wheel Type/Subsystem/Subsystem1/Enabled Subsystem/Average/Subsystem/Enabled Subsystem/If Action Subsystem1/Subsystem ==
  Action Port : ActionPort
  Increament_Wheel1 : Subsystem  Priority=1
      settings: AttributesFormatString=Priority = %<Priority>
  Selecting_threshold : Subsystem  Priority=2
      settings: AttributesFormatString=Priority = %<Priority>  RTWFcnNameOpts=Use subsystem name

== system Mdl_Dim/Mdl_Dim_Task_sys/Subsystem/Input_Process/Thumb Wheel Type/Subsystem/Subsystem1/Enabled Subsystem/Average/Subsystem/Enabled Subsystem/If Action Subsystem/If Action Subsystem1/Increament_Wheel ==
  Process_Step : Subsystem  Priority=1  RTWFcnName=Up_Process_Step
      settings: AttributesFormatString=Priority = %<Priority>  RTWSystemCode=Nonreusable function  RTWFcnNameOpts=User specified
  Subsystem : Subsystem  Commented=on
  Update_Step : Subsystem  Priority=2
      settings: AttributesFormatString=Priority = %<Priority>

== system Mdl_Dim/Mdl_Dim_Task_sys/Subsystem/Input_Process/Thumb Wheel Type/Subsystem/Subsystem1/Enabled Subsystem/Average/Subsystem/Enabled Subsystem/If Action Subsystem/If Action Subsystem1/Selecting_threshold ==
  Add : Sum
  Add1 : Sum  Inputs=+-
  Compare To Constant : simulink/Logic and Bit Operations/Compare To Constant  relop=<  const=POS_MAX  OutDataTypeStr=boolean
  Constant : Constant  Value=WHEEL_INCREAMENT
  Constant1 : Constant  Value=WHEEL_INCREAMENT
  Constant2 : Constant  Value=l_Wheel_Up_ParamArray  OutDataTypeStr=Inherit: Inherit via back propagation
  Constant3 : Constant  Value=l_Wheel_Down_ParamArray  OutDataTypeStr=Inherit: Inherit via back propagation
  Data Store Read{1..4} (4 alike) : DataStoreRead  DataStoreName=l_Wheel_Position_u8  IndexOptions=Index vector (dialog)  Indices=1  OutputSizes=1
  Data Store Write1 : DataStoreWrite  DataStoreName=l_Positionthreshhold_Up  IndexOptions=Index vector (dialog)  Indices=1  OutputSizes=1
  Data Store Write2 : DataStoreWrite  DataStoreName=l_Positionthreshhold_Down  IndexOptions=Index vector (dialog)  Indices=1  OutputSizes=1
  Selector : Selector  IndexMode=Zero-based  InputPortWidth=22  IndexOptions=Index vector (port)  Indices=[1 3]  OutputSizes=1
  Selector1 : Selector  IndexMode=Zero-based  InputPortWidth=22  IndexOptions=Index vector (port)  Indices=[1 3]  OutputSizes=1
  Switch : Switch  Criteria=u2 ~= 0  SaturateOnIntegerOverflow=off  InputSameDT=off
  wires:
  Data Store Read1/1 -> Add/1
  Constant/1 -> Add/2
  Selector/1 -> Data Store Write1/1
  Constant2/1 -> Selector/1
  Add1/1 -> Selector1/2
  Constant3/1 -> Selector1/1
  Selector1/1 -> Data Store Write2/1
  Constant1/1 -> Add1/2
  Data Store Read3/1 -> Add1/1
  Data Store Read2/1 -> Compare To Constant/1
  Compare To Constant/1 -> Switch/2
  Add/1 -> Switch/1
  Data Store Read4/1 -> Switch/3
  Switch/1 -> Selector/2

== system Mdl_Dim/Mdl_Dim_Task_sys/Subsystem/Input_Process/Thumb Wheel Type/Subsystem/Subsystem1/Enabled Subsystem/Average/Subsystem/Enabled Subsystem/If Action Subsystem1/Subsystem/Increament_Wheel1 ==
  Add1 : Sum  Commented=on  Inputs=+-  OutDataTypeStr=uint8
  Assignment_Step : Subsystem  Priority=2
      settings: AttributesFormatString=Priority = %<Priority>
  Constant1 : Constant  Commented=on  Value=WHEEL_INCREAMENT
  Data Store Read3 : DataStoreRead  Commented=on  DataStoreName=l_Wheel_Position_u8  IndexOptions=Index vector (dialog)  Indices=1  OutputSizes=1
  Data Store Write : DataStoreWrite  Commented=on  DataStoreName=l_Wheel_Position_u8  IndexOptions=Index vector (dialog)  Indices=1  OutputSizes=1
  Process_Step : Subsystem  Priority=1  TreatAsAtomicUnit=on  RTWFcnName=Down_Process_Step
      settings: AttributesFormatString=Priority = %<Priority>  RTWSystemCode=Nonreusable function  RTWFcnNameOpts=User specified
  wires:
  Add1/1 -> Data Store Write/1
  Constant1/1 -> Add1/2
  Data Store Read3/1 -> Add1/1

== system Mdl_Dim/Mdl_Dim_Task_sys/Subsystem/Input_Process/Thumb Wheel Type/Subsystem/Subsystem1/Enabled Subsystem/Average/Subsystem/Enabled Subsystem/If Action Subsystem1/Subsystem/Selecting_threshold ==
  Add : Sum
  Add1 : Sum  Inputs=+-
  Compare To Constant1 : simulink/Logic and Bit Operations/Compare To Constant  relop=>  const=POS_MIN  OutDataTypeStr=boolean
  Constant : Constant  Value=WHEEL_INCREAMENT
  Constant1 : Constant  Value=WHEEL_INCREAMENT
  Constant4 : Constant  Value=l_Wheel_Up_ParamArray  OutDataTypeStr=Inherit: Inherit via back propagation
  Constant5 : Constant  Value=l_Wheel_Down_ParamArray  OutDataTypeStr=Inherit: Inherit via back propagation
  Data Store Read{1..4} (4 alike) : DataStoreRead  DataStoreName=l_Wheel_Position_u8  IndexOptions=Index vector (dialog)  Indices=1  OutputSizes=1
  Data Store Write1 : DataStoreWrite  DataStoreName=l_Positionthreshhold_Up  IndexOptions=Index vector (dialog)  Indices=1  OutputSizes=1
  Data Store Write2 : DataStoreWrite  DataStoreName=l_Positionthreshhold_Down  IndexOptions=Index vector (dialog)  Indices=1  OutputSizes=1
  Selector : Selector  IndexMode=Zero-based  InputPortWidth=22  IndexOptions=Index vector (port)  Indices=[1 3]  OutputSizes=1
  Selector1 : Selector  IndexMode=Zero-based  InputPortWidth=22  IndexOptions=Index vector (port)  Indices=[1 3]  OutputSizes=1
  Switch : Switch  Criteria=u2 ~= 0  SaturateOnIntegerOverflow=off  InputSameDT=off
  wires:
  Data Store Read1/1 -> Add/1
  Constant/1 -> Add/2
  Selector/1 -> Data Store Write1/1
  Constant4/1 -> Selector/1
  Constant5/1 -> Selector1/1
  Selector1/1 -> Data Store Write2/1
  Constant1/1 -> Add1/2
  Data Store Read3/1 -> Add1/1
  Add/1 -> Selector/2
  Data Store Read2/1 -> Compare To Constant1/1
  Compare To Constant1/1 -> Switch/2
  Add1/1 -> Switch/1
  Data Store Read4/1 -> Switch/3
  Switch/1 -> Selector1/2

== system Mdl_Dim/Mdl_Dim_Task_sys/Subsystem/Input_Process/Thumb Wheel Type/Subsystem/Subsystem1/Enabled Subsystem/Average/Subsystem/Enabled Subsystem/If Action Subsystem/If Action Subsystem1/Increament_Wheel/Process_Step ==
  Chart1 : Stateflow chart  TreatAsAtomicUnit=on  RTWFcnName=Up_Process_Step
      settings: RTWSystemCode=Nonreusable function  RTWFcnNameOpts=User specified

== system Mdl_Dim/Mdl_Dim_Task_sys/Subsystem/Input_Process/Thumb Wheel Type/Subsystem/Subsystem1/Enabled Subsystem/Average/Subsystem/Enabled Subsystem/If Action Subsystem/If Action Subsystem1/Increament_Wheel/Subsystem ==
  Add1 : Sum  Commented=on  OutDataTypeStr=uint8
  Constant1 : Constant  Commented=on  Value=WHEEL_INCREAMENT
  Data Store Read3 : DataStoreRead  Commented=on  DataStoreName=l_Wheel_Position_u8  IndexOptions=Index vector (dialog)  Indices=1  OutputSizes=1
  Data Store Write : DataStoreWrite  Commented=on  DataStoreName=l_Wheel_Position_u8  IndexOptions=Index vector (dialog)  Indices=1  OutputSizes=1
  For Iterator Subsystem : Subsystem  Commented=on  TreatAsAtomicUnit=on
  wires:
  Constant1/1 -> Add1/2
  Data Store Read3/1 -> Add1/1
  Add1/1 -> Data Store Write/1

== system Mdl_Dim/Mdl_Dim_Task_sys/Subsystem/Input_Process/Thumb Wheel Type/Subsystem/Subsystem1/Enabled Subsystem/Average/Subsystem/Enabled Subsystem/If Action Subsystem/If Action Subsystem1/Increament_Wheel/Update_Step ==
  Data Store Read : DataStoreRead  DataStoreName=l_Wheel_Position_u8  IndexOptions=Index vector (dialog)  Indices=1  OutputSizes=1
  Data Store Write1 : DataStoreWrite  DataStoreName=l_Wheel_Position_Temp_u8  IndexOptions=Index vector (dialog)  Indices=1  OutputSizes=1
  wires:
  Data Store Read/1 -> Data Store Write1/1

== system Mdl_Dim/Mdl_Dim_Task_sys/Subsystem/Input_Process/Thumb Wheel Type/Subsystem/Subsystem1/Enabled Subsystem/Average/Subsystem/Enabled Subsystem/If Action Subsystem1/Subsystem/Increament_Wheel1/Assignment_Step ==
  Data Store Read : DataStoreRead  DataStoreName=l_Wheel_Position_u8  IndexOptions=Index vector (dialog)  Indices=1  OutputSizes=1
  Data Store Write1 : DataStoreWrite  DataStoreName=l_Wheel_Position_Temp_u8  IndexOptions=Index vector (dialog)  Indices=1  OutputSizes=1
  wires:
  Data Store Read/1 -> Data Store Write1/1

== system Mdl_Dim/Mdl_Dim_Task_sys/Subsystem/Input_Process/Thumb Wheel Type/Subsystem/Subsystem1/Enabled Subsystem/Average/Subsystem/Enabled Subsystem/If Action Subsystem1/Subsystem/Increament_Wheel1/Process_Step ==
  Chart : Stateflow chart  TreatAsAtomicUnit=on

== system Mdl_Dim/Mdl_Dim_Task_sys/Subsystem/Input_Process/Thumb Wheel Type/Subsystem/Subsystem1/Enabled Subsystem/Average/Subsystem/Enabled Subsystem/If Action Subsystem/If Action Subsystem1/Increament_Wheel/Subsystem/For Iterator Subsystem ==
  Add : Sum
  Constant : Constant  Value=VAL_ONE
  Constant1 : Constant  Value=VAL_ZERO
  Constant2 : Constant  Value=l_Wheel_Up_ParamArray  OutDataTypeStr=Inherit: Inherit via back propagation
  Data Store Memory : DataStoreMemory  DataStoreName=i  ReadBeforeWriteMsg=warning  WriteAfterWriteMsg=warning  WriteAfterReadMsg=warning  ShowAdditionalParam=off
  Data Store Read : DataStoreRead  DataStoreName=l_Wheel_Position_u8  IndexOptions=Index vector (dialog)  Indices=1  OutputSizes=1
  Data Store Read1 : DataStoreRead  DataStoreName=i  IndexOptions=Index vector (dialog)  Indices=1  OutputSizes=1
  Data Store Read6 : DataStoreRead  DataStoreName=l_Wheel_AveVol_u32  IndexOptions=Index vector (dialog)  Indices=1  OutputSizes=1
  Data Store Write : DataStoreWrite  DataStoreName=i  IndexOptions=Index vector (dialog)  Indices=1  OutputSizes=1
  Data Store Write1 : DataStoreWrite  DataStoreName=i  IndexOptions=Index vector (dialog)  Indices=1  OutputSizes=1
  Data Store Write2 : DataStoreWrite  DataStoreName=l_Wheel_Position_u8  IndexOptions=Index vector (dialog)  Indices=1  OutputSizes=1
  For Iterator : ForIterator  ResetStates=reset  IterationLimit=21  ExternalIncrement=on  IndexMode=Zero-based  IterationVariableDataType=int8
  GreaterThan : RelationalOperator  Operator=>  OutDataTypeStr=boolean  RndMeth=Simplest  InputSameDT=off
  Selector : Selector  IndexMode=Zero-based  InputPortWidth=22  IndexOptions=Index vector (port)  Indices=[1 3]  OutputSizes=1
  Switch : Switch  Criteria=u2 ~= 0  SaturateOnIntegerOverflow=off  InputSameDT=off
  wires:
  Constant2/1 -> Selector/1
  Add/1 -> Selector/2
  For Iterator/1 -> [position], Add/1
  Constant/1 -> Add/2
  Selector/1 -> GreaterThan/1
  GreaterThan/1 -> Switch/2
  Switch/1 -> Data Store Write2/1
  Data Store Read6/1 -> GreaterThan/2
  [position] -> Switch/1
  Data Store Read/1 -> Switch/3
  Data Store Read1/1 -> For Iterator/1
  Constant1/1 -> Data Store Write1/1

== stateflow chart Mdl_Dim/Mdl_Dim_Task_sys/Subsystem/Input_Process/Thumb Wheel Type/Subsystem/Subsystem1/Enabled Subsystem/Average/Subsystem/Enabled Subsystem/If Action Subsystem1/Subsystem/Increament_Wheel1/Process_Step/Chart ==
  (default) -> (junction 2)
  (junction 1) -> (junction 2) [order 1] : [(l_Wheel_Position_u8 ~= 0) && (l_Wheel_AveVol_u32 < l_Wheel_Down_ParamArray[l_Wheel_Position_u8 - VAL_ONE])]
  (junction 2) -> (junction 1) [order 1] : [l_Wheel_AveVol_u32 <= l_Wheel_Down_ParamArray[l_Wheel_Position_u8]]
      | {l_Wheel_Position_u8 = l_Wheel_Position_u8 - VAL_ONE}
  (junction 11) -> (junction 1)
  (junction 2) -> (junction 11) [order 2]
  (junction 1) -> (junction 24) [order 2]
  data: l_Wheel_AveVol_u32 data_store_memory; l_Wheel_Position_u8 data_store_memory; VAL_ONE parameter; l_Wheel_Down_ParamArray parameter

== stateflow chart Mdl_Dim/Mdl_Dim_Task_sys/Subsystem/Input_Process/Thumb Wheel Type/Subsystem/Subsystem1/Enabled Subsystem/Average/Subsystem/Enabled Subsystem/If Action Subsystem/If Action Subsystem1/Increament_Wheel/Process_Step/Chart1 ==
  (default) -> (junction 2)
  (junction 1) -> (junction 2) [order 1] : [(l_Wheel_Position_u8 < POS_MAX ) && (l_Wheel_AveVol_u32 >= l_Wheel_Up_ParamArray[l_Wheel_Position_u8 + VAL_ONE])]
  (junction 2) -> (junction 1) [order 1] : [l_Wheel_AveVol_u32 >= l_Wheel_Up_ParamArray[l_Wheel_Position_u8 + VAL_ONE]]{l_Wheel_Position_u8 = l_Wheel_Position_u8 + VAL_ONE}
  (junction 11) -> (junction 1)
  (junction 2) -> (junction 11) [order 2]
  (junction 1) -> (junction 24) [order 2]
  data: l_Wheel_AveVol_u32 data_store_memory; l_Wheel_Position_u8 data_store_memory; POS_MAX parameter; VAL_ONE parameter; l_Wheel_Up_ParamArray parameter

== matlab function Mdl_Dim/Mdl_Dim_Task_sys/Subsystem/Input_Process/Subsystem/TAIL_Status_Processing ==
  data: Ignitionmode input; TailCANstatus input; TailCanVal input; Appmode input; TailStatus output uint8; NETWORK_NORMAL parameter; RTE_E_NEVER_RECEIVED parameter; PrevTailStsVal input; CAN_VAL_ON parameter; CAN_VAL_OFF parameter; RTE_E_MAX_AGE_EXCEEDED parameter; IgnOn parameter; NETWORK_SLEEP parameter; NETWORK_STANDALONE parameter; CAN_COMUN_ACTIVE parameter; VAL_OFF parameter; VAL_ON parameter; TRUE parameter; FALSE parameter
function TailStatus = fcn(Ignitionmode, TailCANstatus, TailCanVal, Appmode, NETWORK_NORMAL, RTE_E_NEVER_RECEIVED, PrevTailStsVal, CAN_VAL_ON, CAN_VAL_OFF, RTE_E_MAX_AGE_EXCEEDED, IgnOn, NETWORK_SLEEP, NETWORK_STANDALONE, CAN_COMUN_ACTIVE, VAL_OFF, VAL_ON, TRUE, FALSE)

aVarTruthTableCondition_1 = false;
aVarTruthTableCondition_2 = false;
aVarTruthTableCondition_3 = false;
aVarTruthTableCondition_4 = false;



aVarTruthTableCondition_1 = logical(((Appmode == NETWORK_SLEEP) || ((Appmode == NETWORK_NORMAL) &&  (TailCANstatus == RTE_E_MAX_AGE_EXCEEDED) && (Ignitionmode == VAL_OFF))));

% condition 1

aVarTruthTableCondition_2 = logical(((Appmode == NETWORK_STANDALONE) || ((Appmode == NETWORK_NORMAL) && ((TailCANstatus == RTE_E_NEVER_RECEIVED) || ((TailCANstatus == RTE_E_MAX_AGE_EXCEEDED)  && (Ignitionmode == VAL_ON))))));

% condition 2

aVarTruthTableCondition_3 = logical(( (Appmode == NETWORK_NORMAL) && (TailCANstatus == CAN_COMUN_ACTIVE) && (TailCanVal ==CAN_VAL_OFF) ));

% condition 3

aVarTruthTableCondition_4 = logical(( (Appmode == NETWORK_NORMAL) && (TailCANstatus == CAN_COMUN_ACTIVE) && (TailCanVal == CAN_VAL_ON) ));

if (aVarTruthTableCondition_1)
    aFcnTruthTableAction_2();
elseif (aVarTruthTableCondition_2)
    aFcnTruthTableAction_1();
elseif (aVarTruthTableCondition_3)
    aFcnTruthTableAction_2();
elseif (aVarTruthTableCondition_4)
    aFcnTruthTableAction_3();
else % Default
    aFcnTruthTableAction_2();
end

function aFcnTruthTableAction_1()

    % Example action 1 called from D1, D4 & D5 column in condition table

    TailStatus = PrevTailStsVal;

function aFcnTruthTableAction_2()

    % Example action 2 called from D2 &D6 column in condition table

    TailStatus = CAN_VAL_OFF;

function aFcnTruthTableAction_3()

    % Example action 2 called from D3 column in condition table

    TailStatus = CAN_VAL_ON;
